simulink model "MPC"  (R2024b)
settings: Solver=ode4  StartTime=0.0  StopTime=tsim  FixedStep=baseRate  RelTol=1e-6  AbsTol=1e-6
values from neighbouring files (symbols this model uses):
  C = [cos(theta), -sin(theta) ... (first row only)    [Run_Initializer.m]    (also in plotBatch.m = quat2Rotm(q','scalarFirst'))
  camera_FOV = 40*d2r    (= 0.698131700798)    [Run_Initializer.m]
  camera_offset = [0.145, 0.087]'    [Run_Initializer.m]
  docking_face = [0 1]'    [Run_Initializer.m]
  docking_offset = [0 0 0]'    [Run_Initializer.m]
  eta = 0.7    [Run_Initializer.m]
  F_t = [kron(eye(N_h),  [zeros(2,3), eye(2), zeros(2,4)]) ... (first row only)    [Run_Initializer.m]
  f_t = [kron(ones(N_h, 1), [xLength yLength]' - edge_buffer) ... (first row only)    [Run_Initializer.m]
  F_u = [kron(eye(N_h),  [eye(3), zeros(3,6)]) ... (first row only)    [Run_Initializer.m]
  f_u = kron(ones(2*N_h, 1), u_max')    [Run_Initializer.m]
  F_v = [kron(eye(N_h),  [zeros(1,5), 1, zeros(1,3)]) ... (first row only)    [Run_Initializer.m]
  gamma = 0.95    [Run_Initializer.m]
  Gamma1_el = 0.12    [Run_Initializer.m]
  Gamma1_sh = 0.005    [Run_Initializer.m]
  Gamma1_wr = 0.025    [Run_Initializer.m]
  Gamma2_el = 5    [Run_Initializer.m]
  Gamma2_sh = 5    [Run_Initializer.m]
  Gamma2_wr = 5    [Run_Initializer.m]
  Gamma3_el = 10    [Run_Initializer.m]
  Gamma3_sh = 40    [Run_Initializer.m]
  Gamma3_wr = 40    [Run_Initializer.m]
  Gamma4_el = 0.039    [Run_Initializer.m]
  Gamma4_sh = 0.015    [Run_Initializer.m]
  Gamma4_wr = 0.029    [Run_Initializer.m]
  Gamma5_el = 800    [Run_Initializer.m]
  Gamma5_sh = 800    [Run_Initializer.m]
  Gamma5_wr = 800    [Run_Initializer.m]
  Gamma6_el = 0.000001    (= 1e-06)    [Run_Initializer.m]
  Gamma6_sh = 0.005    [Run_Initializer.m]
  Gamma6_wr = 0.02    [Run_Initializer.m]
  H = kron(eye(N_h), [R, zeros(3,6); zeros(6,3), Q])    [Run_Initializer.m]
  IBLACK = 0.1996    [unpackData.m]
  IRED = 0.1982    [unpackData.m]
  J = sum(wp*posErr + wt*angErr)    [find_transformation.m]
  Kd_elarm = 0.8    [Run_Initializer.m]
  Kd_sharm = 1.0    (= 1)    [Run_Initializer.m]
  Kd_wrarm = 0.6    [Run_Initializer.m]
  Kp_elarm = 1.2    [Run_Initializer.m]
  Kp_sharm = 1.5    [Run_Initializer.m]
  Kp_wrarm = 1.0    (= 1)    [Run_Initializer.m]
  m = m + 5    (= 4)    [unpackData.m]
  M = diag([1/m; 1/m; 1/I])    [unpackData.m]
  maxd = [d1 ... (first row only)    [Run_Initializer.m]
  mBLACK = 11.3620    (= 11.362)    [unpackData.m]
  mRED = 11.2970    (= 11.297)    [unpackData.m]
  N = size(rel,1)    [plotBatch.m]    (also in unpackData.m = 0)
  p = [0 obj.pos(k,:)]    [SparseState6DOF.m]
  PDQ = blkdiag(20*eye(3),eye(3), 20*eye(3),eye(3))    [Run_Initializer.m]
  PQ = blkdiag(20*eye(6),eye(6))    [Run_Initializer.m]
  PR = blkdiag(20*eye(3), eye(6), 0.0001*eye(3))    [Run_Initializer.m]
  PWMFreq = 5    [Run_Initializer.m]
  Q = diag([100 100 100 300 300 300])    [Run_Initializer.m]    (also in unpackData.m = blkdiag(0.0001*eye(2), 0.00001))
  R = diag([200 200 200])    [Run_Initializer.m]    (also in plotBatch.m = C3(yaw); unpackData.m = diag([6;6;6]))
  r_hold_obs = 1.1*sqrt(2)*0.3.*[1 1]    [Run_Initializer.m]
  r_hold_tar_min = [0.8; (0.3+0.05)]    [Run_Initializer.m]
  rho = 0.98    [Run_Initializer.m]
  T_d = 2    [Run_Initializer.m]
  T_max = 0.15    [Run_Initializer.m]
  Tz_lim_elarm = .1    (= 0.1)    [Run_Initializer.m]
  Tz_lim_sharm = .1    (= 0.1)    [Run_Initializer.m]
  Tz_lim_wrarm = .1    (= 0.1)    [Run_Initializer.m]
  use_LOS_constr = 1    [Run_Initializer.m]
  use_table_constr = 1    [Run_Initializer.m]
  x_BLACK_0 = [(1/3)*xLength (1/3)*yLength-0.2 280*d2r 0.01 0.005 1.88*d2r]'    [Run_Initializer.m]
  x_BLUE_0 = [0 0 0 0 0 0]'    [Run_Initializer.m]
  zeta = 10*d2r    (= 0.174532925199)    [Run_Initializer.m]
undefined symbols (not defined in the file or in its folder): a1, a2, a3, alpha, alpha_m, alpha_t, alphas, alphas_t, alphat, Am, b, b0, b1, b2, b3, baseRate, Bm, c, c1, c1t, c2, c2t, Cm, d, dataRate, DiscIntNeverNeededParam, Dm, drop_states_ARM, drop_states_BLACK, drop_states_BLUE, drop_states_RED, epsilon, epsilont, F_black_X_nominal, F_black_Y_nominal, F_blue_X_nominal, F_blue_Y_nominal, F_max, F_red_X_nominal, F_red_Y_nominal, F_thrusters_BLACK, F_thrusters_BLUE, F_thrusters_RED, gamma_I, gamma_I_t, gamma_P, gamma_P_t, home_states_BLACK, home_states_BLUE, home_states_RED, IBLUE, IDIST, IEE, init_states_BLACK, init_states_BLUE, init_states_RED, IPROX, k, K, k1 ... (+62)
libraries: simulink x33, nvidiaSharedBlocks x13, slpidlib x6, MainLibrary x5, dspsigops x3, dspinverses x3, nvidiaIMUSensorslib x1
(part 6 of 12)

== system MPC/3 - Navigation/Subsystem/QMEKF ==
  Data Store Read : DataStoreRead  DataStoreName=dt  IndexOptions=Index vector (dialog)  Indices=1  OutputSizes=1
  Data Store Read1 : DataStoreRead  DataStoreName=Red_q  IndexOptions=Index vector (dialog)  Indices=1  OutputSizes=1
  Data Store Read2 : DataStoreRead  DataStoreName=Red_x  IndexOptions=Index vector (dialog)  Indices=1  OutputSizes=1
  Data Store Read3 : DataStoreRead  DataStoreName=Vis_q  IndexOptions=Index vector (dialog)  Indices=1  OutputSizes=1
  Data Store Read4 : DataStoreRead  DataStoreName=Vis_x  IndexOptions=Index vector (dialog)  Indices=1  OutputSizes=1
  Data Store Write1 : DataStoreWrite  DataStoreName=QMEKFerror  IndexOptions=Index vector (dialog)  Indices=1  OutputSizes=1
  Data Store Write17 : DataStoreWrite  DataStoreName=QMEKFx  IndexOptions=Index vector (dialog)  Indices=1  OutputSizes=1
  Data Store Write18 : DataStoreWrite  DataStoreName=QMEKFP  IndexOptions=Index vector (dialog)  Indices=1  OutputSizes=1
  Data Store Write19 : DataStoreWrite  DataStoreName=QMEKFt  IndexOptions=Index vector (dialog)  Indices=1  OutputSizes=1
  Data Store Write2 : DataStoreWrite  DataStoreName=QMEKFNIS  IndexOptions=Index vector (dialog)  Indices=1  OutputSizes=1
  Delay : Delay  DelayLength=1  InitialCondition=PQ
  Delay1 : Delay  DelayLength=1  InitialCondition=[1;zeros(12,1)]
  MATLAB Function : MATLAB Function  TreatAsAtomicUnit=on
  MATLAB Function1 : MATLAB Function  TreatAsAtomicUnit=on
  wires:
  Delay/1 -> MATLAB Function1/7(P_prev)
  MATLAB Function1/2(P_est) -> Delay/1, Data Store Write18/1
  Delay1/1 -> MATLAB Function1/6(x_prev)
  MATLAB Function1/1(x_est) -> MATLAB Function/1(u), Delay1/1
  MATLAB Function1/3(compT) -> Data Store Write19/1
  Data Store Read/1 -> MATLAB Function1/1(dt)
  Data Store Read1/1 -> MATLAB Function1/2(RED_quat)
  Data Store Read2/1 -> MATLAB Function1/3(RED_x)
  Data Store Read3/1 -> MATLAB Function1/4(BLACK_q)
  Data Store Read4/1 -> MATLAB Function1/5(BLACK_x)
  MATLAB Function/1(out) -> Data Store Write17/1
  MATLAB Function1/5(NIS) -> Data Store Write2/1  "NIS"
  MATLAB Function1/4(y) -> Data Store Write1/1

== system MPC/3 - Navigation/Subsystem/RMEKF ==
  Data Store Read : DataStoreRead  DataStoreName=dt  IndexOptions=Index vector (dialog)  Indices=1  OutputSizes=1
  Data Store Read15 : DataStoreRead  DataStoreName=Vis_R  IndexOptions=Index vector (dialog)  Indices=1  OutputSizes=1
  Data Store Read2 : DataStoreRead  DataStoreName=Red_x  IndexOptions=Index vector (dialog)  Indices=1  OutputSizes=1
  Data Store Read3 : DataStoreRead  DataStoreName=Red_q  IndexOptions=Index vector (dialog)  Indices=1  OutputSizes=1
  Data Store Read4 : DataStoreRead  DataStoreName=Vis_x  IndexOptions=Index vector (dialog)  Indices=1  OutputSizes=1
  Data Store Write1 : DataStoreWrite  DataStoreName=RMEKFR  IndexOptions=Index vector (dialog)  Indices=1  OutputSizes=1
  Data Store Write17 : DataStoreWrite  DataStoreName=RMEKFx  IndexOptions=Index vector (dialog)  Indices=1  OutputSizes=1
  Data Store Write18 : DataStoreWrite  DataStoreName=RMEKFP  IndexOptions=Index vector (dialog)  Indices=1  OutputSizes=1
  Data Store Write19 : DataStoreWrite  DataStoreName=RMEKFt  IndexOptions=Index vector (dialog)  Indices=1  OutputSizes=1
  Data Store Write2 : DataStoreWrite  DataStoreName=RMEKFerror  IndexOptions=Index vector (dialog)  Indices=1  OutputSizes=1
  Data Store Write6 : DataStoreWrite  DataStoreName=RMEKFNIS  IndexOptions=Index vector (dialog)  Indices=1  OutputSizes=1
  Delay : Delay  DelayLength=1  InitialCondition=PR
  Delay1 : Delay  DelayLength=1  InitialCondition=zeros(9,1)
  Delay2 : Delay  DelayLength=1  InitialCondition=eye(3)
  MATLAB Function : MATLAB Function  TreatAsAtomicUnit=on
  MATLAB Function1 : MATLAB Function  TreatAsAtomicUnit=on
  MATLAB Function11 : MATLAB Function  TreatAsAtomicUnit=on
  wires:
  Delay/1 -> MATLAB Function1/8(P_prev)
  MATLAB Function1/3(P_est) -> Delay/1, Data Store Write18/1
  Delay1/1 -> MATLAB Function1/6(x_prev)
  MATLAB Function1/1(x_est) -> Delay1/1, MATLAB Function/1(x)
  MATLAB Function1/4(compT) -> Data Store Write19/1
  Data Store Read/1 -> MATLAB Function1/1(dt)
  Data Store Read3/1 -> MATLAB Function1/2(RED_yaw)
  Data Store Read2/1 -> MATLAB Function1/3(RED_x)
  Data Store Read15/1 -> MATLAB Function1/4(VIS_R)
  Data Store Read4/1 -> MATLAB Function1/5(VIS_x)
  MATLAB Function1/2(Rot_est) -> Delay2/1, Data Store Write1/1, MATLAB Function11/1(u)
  Delay2/1 -> MATLAB Function1/7(Rot_prev)
  MATLAB Function11/1(y) -> MATLAB Function/2(q)  "q"
  MATLAB Function/1(out) -> Data Store Write17/1
  MATLAB Function1/6(NIS) -> Data Store Write6/1  "NIS"
  MATLAB Function1/5(y) -> Data Store Write2/1

== system MPC/3 - Navigation/Subsystem/Representations ==
  u : Inport
  MATLAB Function : MATLAB Function  TreatAsAtomicUnit=on
  dq : Outport
  q : Outport  Port=2
  R : Outport  Port=3
  x : Outport  Port=4
  v : Outport  Port=5
  w : Outport  Port=6
  yaw : Outport  Port=7
  wires:
  u/1 -> MATLAB Function/1(u)
  MATLAB Function/1(dq) -> dq/1
  MATLAB Function/2(q) -> q/1
  MATLAB Function/3(R) -> R/1
  MATLAB Function/4(x) -> x/1
  MATLAB Function/5(v) -> v/1
  MATLAB Function/6(w) -> w/1
  MATLAB Function/7(yaw) -> yaw/1

== system MPC/3 - Navigation/Subsystem/Representations1 ==
  u : Inport
  MATLAB Function : MATLAB Function  TreatAsAtomicUnit=on
  dq : Outport
  q : Outport  Port=2
  R : Outport  Port=3
  x : Outport  Port=4
  v : Outport  Port=5
  w : Outport  Port=6
  yaw : Outport  Port=7
  wires:
  u/1 -> MATLAB Function/1(u)
  MATLAB Function/1(dq) -> dq/1
  MATLAB Function/2(q) -> q/1
  MATLAB Function/3(R) -> R/1
  MATLAB Function/4(x) -> x/1
  MATLAB Function/5(v) -> v/1
  MATLAB Function/6(w) -> w/1
  MATLAB Function/7(yaw) -> yaw/1

== system MPC/3 - Navigation/Subsystem/STDQMEKF ==
  Data Store Read : DataStoreRead  DataStoreName=dt  IndexOptions=Index vector (dialog)  Indices=1  OutputSizes=1
  Data Store Read1 : DataStoreRead  DataStoreName=Vis_dq  IndexOptions=Index vector (dialog)  Indices=1  OutputSizes=1
  Data Store Read2 : DataStoreRead  DataStoreName=Red_dq  IndexOptions=Index vector (dialog)  Indices=1  OutputSizes=1
  Data Store Write1 : DataStoreWrite  DataStoreName=STDQMEKFerror  IndexOptions=Index vector (dialog)  Indices=1  OutputSizes=1
  Data Store Write17 : DataStoreWrite  DataStoreName=STDQMEKFx  IndexOptions=Index vector (dialog)  Indices=1  OutputSizes=1
  Data Store Write18 : DataStoreWrite  DataStoreName=STDQMEKFP  IndexOptions=Index vector (dialog)  Indices=1  OutputSizes=1
  Data Store Write19 : DataStoreWrite  DataStoreName=STDQMEKFt  IndexOptions=Index vector (dialog)  Indices=1  OutputSizes=1
  Data Store Write2 : DataStoreWrite  DataStoreName=STDQMEKFNIS  IndexOptions=Index vector (dialog)  Indices=1  OutputSizes=1
  Delay : Delay  DelayLength=1  InitialCondition=PDQ
  Delay1 : Delay  DelayLength=1  InitialCondition=[1;zeros(13,1)]
  Delay2 : Delay  DelayLength=1  InitialCondition=zeros(6)
  MATLAB Function1 : MATLAB Function  TreatAsAtomicUnit=on
  MATLAB Function3 : MATLAB Function  TreatAsAtomicUnit=on
  wires:
  Delay/1 -> MATLAB Function1/5(P_prev)
  Delay1/1 -> MATLAB Function1/4(x_prev)
  MATLAB Function1/1(x_est) -> Delay1/1, MATLAB Function3/1(u)
  Data Store Read/1 -> MATLAB Function1/1(dt)
  MATLAB Function1/6(V_est) -> Delay2/1
  Delay2/1 -> MATLAB Function1/6(V_prev)
  Data Store Read2/1 -> MATLAB Function1/2(RED_dq)
  Data Store Read1/1 -> MATLAB Function1/3(VIS_dq)
  MATLAB Function1/3(compT) -> Data Store Write19/1
  MATLAB Function3/1(x) -> Data Store Write17/1
  MATLAB Function1/2(P_est) -> Delay/1, Data Store Write18/1
  MATLAB Function1/4(y) -> Data Store Write1/1
  MATLAB Function1/5(NIS) -> Data Store Write2/1

== system MPC/3 - Navigation/Subsystem/STDQMEKF1 ==
  Data Store Read : DataStoreRead  DataStoreName=dt  IndexOptions=Index vector (dialog)  Indices=1  OutputSizes=1
  Data Store Read1 : DataStoreRead  DataStoreName=Vis_dq  IndexOptions=Index vector (dialog)  Indices=1  OutputSizes=1
  Data Store Read2 : DataStoreRead  DataStoreName=Red_dq  IndexOptions=Index vector (dialog)  Indices=1  OutputSizes=1
  Data Store Write1 : DataStoreWrite  DataStoreName=STDQMEKFerror2  IndexOptions=Index vector (dialog)  Indices=1  OutputSizes=1
  Data Store Write17 : DataStoreWrite  DataStoreName=STDQMEKFx2  IndexOptions=Index vector (dialog)  Indices=1  OutputSizes=1
  Data Store Write18 : DataStoreWrite  DataStoreName=STDQMEKFP2  IndexOptions=Index vector (dialog)  Indices=1  OutputSizes=1
  Data Store Write19 : DataStoreWrite  DataStoreName=STDQMEKFt2  IndexOptions=Index vector (dialog)  Indices=1  OutputSizes=1
  Data Store Write2 : DataStoreWrite  DataStoreName=STDQMEKFNIS2  IndexOptions=Index vector (dialog)  Indices=1  OutputSizes=1
  Delay : Delay  DelayLength=1  InitialCondition=PDQ
  Delay1 : Delay  DelayLength=1  InitialCondition=[1;zeros(13,1)]
  Delay2 : Delay  DelayLength=1  InitialCondition=zeros(6)
  MATLAB Function1 : MATLAB Function  TreatAsAtomicUnit=on
  MATLAB Function3 : MATLAB Function  TreatAsAtomicUnit=on
  wires:
  Delay/1 -> MATLAB Function1/5(P_prev)
  Delay1/1 -> MATLAB Function1/4(x_prev)
  MATLAB Function1/1(x_est) -> Delay1/1, MATLAB Function3/1(u)
  Data Store Read/1 -> MATLAB Function1/1(dt)
  MATLAB Function1/6(V_est) -> Delay2/1
  Delay2/1 -> MATLAB Function1/6(V_prev)
  Data Store Read2/1 -> MATLAB Function1/2(RED_dq)
  Data Store Read1/1 -> MATLAB Function1/3(VIS_dq)
  MATLAB Function1/3(compT) -> Data Store Write19/1
  MATLAB Function3/1(x) -> Data Store Write17/1
  MATLAB Function1/2(P_est) -> Delay/1, Data Store Write18/1
  MATLAB Function1/4(y) -> Data Store Write1/1
  MATLAB Function1/5(NIS) -> Data Store Write2/1

== system MPC/3 - Navigation/Subsystem/STQMEKF ==
  Data Store Read : DataStoreRead  DataStoreName=dt  IndexOptions=Index vector (dialog)  Indices=1  OutputSizes=1
  Data Store Read1 : DataStoreRead  DataStoreName=Red_q  IndexOptions=Index vector (dialog)  Indices=1  OutputSizes=1
  Data Store Read2 : DataStoreRead  DataStoreName=Red_x  IndexOptions=Index vector (dialog)  Indices=1  OutputSizes=1
  Data Store Read3 : DataStoreRead  DataStoreName=Vis_q  IndexOptions=Index vector (dialog)  Indices=1  OutputSizes=1
  Data Store Read4 : DataStoreRead  DataStoreName=Vis_x  IndexOptions=Index vector (dialog)  Indices=1  OutputSizes=1
  Data Store Write1 : DataStoreWrite  DataStoreName=STQMEKFerror  IndexOptions=Index vector (dialog)  Indices=1  OutputSizes=1
  Data Store Write17 : DataStoreWrite  DataStoreName=STQMEKFx  IndexOptions=Index vector (dialog)  Indices=1  OutputSizes=1
  Data Store Write18 : DataStoreWrite  DataStoreName=STQMEKFP  IndexOptions=Index vector (dialog)  Indices=1  OutputSizes=1
  Data Store Write19 : DataStoreWrite  DataStoreName=STQMEKFt  IndexOptions=Index vector (dialog)  Indices=1  OutputSizes=1
  Data Store Write2 : DataStoreWrite  DataStoreName=STQMEKFNIS  IndexOptions=Index vector (dialog)  Indices=1  OutputSizes=1
  Delay : Delay  DelayLength=1  InitialCondition=PQ
  Delay1 : Delay  DelayLength=1  InitialCondition=[1;zeros(12,1)]
  Delay2 : Delay  DelayLength=1  InitialCondition=zeros(6)
  MATLAB Function1 : MATLAB Function  TreatAsAtomicUnit=on
  MATLAB Function2 : MATLAB Function  TreatAsAtomicUnit=on
  wires:
  Delay/1 -> MATLAB Function1/7(P_prev)
  MATLAB Function1/2(P_est) -> Delay/1, Data Store Write18/1
  Delay1/1 -> MATLAB Function1/6(x_prev)
  MATLAB Function1/1(x_est) -> MATLAB Function2/1(u), Delay1/1
  Data Store Read/1 -> MATLAB Function1/1(dt)
  Data Store Read1/1 -> MATLAB Function1/2(RED_quat)
  Data Store Read2/1 -> MATLAB Function1/3(RED_x)
  Data Store Read3/1 -> MATLAB Function1/4(BLACK_q)
  Data Store Read4/1 -> MATLAB Function1/5(BLACK_x)
  MATLAB Function1/6(V_est) -> Delay2/1
  Delay2/1 -> MATLAB Function1/8(V_prev)
  MATLAB Function2/1(out) -> Data Store Write17/1
  MATLAB Function1/4(y) -> Data Store Write1/1
  MATLAB Function1/5(NIS) -> Data Store Write2/1  "NIS"
  MATLAB Function1/3(compT) -> Data Store Write19/1

== system MPC/3 - Navigation/Subsystem/STQMEKF1 ==
  Data Store Read : DataStoreRead  DataStoreName=dt  IndexOptions=Index vector (dialog)  Indices=1  OutputSizes=1
  Data Store Read1 : DataStoreRead  DataStoreName=Red_q  IndexOptions=Index vector (dialog)  Indices=1  OutputSizes=1
  Data Store Read2 : DataStoreRead  DataStoreName=Red_x  IndexOptions=Index vector (dialog)  Indices=1  OutputSizes=1
  Data Store Read3 : DataStoreRead  DataStoreName=Vis_q  IndexOptions=Index vector (dialog)  Indices=1  OutputSizes=1
  Data Store Read4 : DataStoreRead  DataStoreName=Vis_x  IndexOptions=Index vector (dialog)  Indices=1  OutputSizes=1
  Data Store Write1 : DataStoreWrite  DataStoreName=STQMEKFerror2  IndexOptions=Index vector (dialog)  Indices=1  OutputSizes=1
  Data Store Write17 : DataStoreWrite  DataStoreName=STQMEKFx2  IndexOptions=Index vector (dialog)  Indices=1  OutputSizes=1
  Data Store Write18 : DataStoreWrite  DataStoreName=STQMEKFP2  IndexOptions=Index vector (dialog)  Indices=1  OutputSizes=1
  Data Store Write19 : DataStoreWrite  DataStoreName=STQMEKFt2  IndexOptions=Index vector (dialog)  Indices=1  OutputSizes=1
  Data Store Write2 : DataStoreWrite  DataStoreName=STQMEKFNIS2  IndexOptions=Index vector (dialog)  Indices=1  OutputSizes=1
  Delay : Delay  DelayLength=1  InitialCondition=PQ
  Delay1 : Delay  DelayLength=1  InitialCondition=[1;zeros(12,1)]
  Delay2 : Delay  DelayLength=1  InitialCondition=zeros(6)
  MATLAB Function1 : MATLAB Function  TreatAsAtomicUnit=on
  MATLAB Function2 : MATLAB Function  TreatAsAtomicUnit=on
  wires:
  Delay/1 -> MATLAB Function1/7(P_prev)
  MATLAB Function1/2(P_est) -> Delay/1, Data Store Write18/1
  Delay1/1 -> MATLAB Function1/6(x_prev)
  MATLAB Function1/1(x_est) -> MATLAB Function2/1(u), Delay1/1
  Data Store Read/1 -> MATLAB Function1/1(dt)
  Data Store Read1/1 -> MATLAB Function1/2(RED_quat)
  Data Store Read2/1 -> MATLAB Function1/3(RED_x)
  Data Store Read3/1 -> MATLAB Function1/4(BLACK_q)
  Data Store Read4/1 -> MATLAB Function1/5(BLACK_x)
  MATLAB Function1/6(V_est) -> Delay2/1
  Delay2/1 -> MATLAB Function1/8(V_prev)
  MATLAB Function2/1(out) -> Data Store Write17/1
  MATLAB Function1/4(y) -> Data Store Write1/1
  MATLAB Function1/5(NIS) -> Data Store Write2/1  "NIS"
  MATLAB Function1/3(compT) -> Data Store Write19/1

== system MPC/3 - Navigation/Subsystem/STRMEKF ==
  Data Store Read : DataStoreRead  DataStoreName=dt  IndexOptions=Index vector (dialog)  Indices=1  OutputSizes=1
  Data Store Read1 : DataStoreRead  DataStoreName=Vis_R  IndexOptions=Index vector (dialog)  Indices=1  OutputSizes=1
  Data Store Read2 : DataStoreRead  DataStoreName=Red_x  IndexOptions=Index vector (dialog)  Indices=1  OutputSizes=1
  Data Store Read3 : DataStoreRead  DataStoreName=Red_q  IndexOptions=Index vector (dialog)  Indices=1  OutputSizes=1
  Data Store Read4 : DataStoreRead  DataStoreName=Vis_x  IndexOptions=Index vector (dialog)  Indices=1  OutputSizes=1
  Data Store Write1 : DataStoreWrite  DataStoreName=STRMEKFR  IndexOptions=Index vector (dialog)  Indices=1  OutputSizes=1
  Data Store Write17 : DataStoreWrite  DataStoreName=STRMEKFx  IndexOptions=Index vector (dialog)  Indices=1  OutputSizes=1
  Data Store Write18 : DataStoreWrite  DataStoreName=STRMEKFP  IndexOptions=Index vector (dialog)  Indices=1  OutputSizes=1
  Data Store Write19 : DataStoreWrite  DataStoreName=STRMEKFt  IndexOptions=Index vector (dialog)  Indices=1  OutputSizes=1
  Data Store Write2 : DataStoreWrite  DataStoreName=STRMEKFerror  IndexOptions=Index vector (dialog)  Indices=1  OutputSizes=1
  Data Store Write6 : DataStoreWrite  DataStoreName=STRMEKFNIS  IndexOptions=Index vector (dialog)  Indices=1  OutputSizes=1
  Delay1 : Delay  DelayLength=1  InitialCondition=zeros(9,1)
  Delay2 : Delay  DelayLength=1  InitialCondition=PR
  Delay3 : Delay  DelayLength=1  InitialCondition=zeros(6)
  Delay4 : Delay  DelayLength=1  InitialCondition=eye(3)
  MATLAB Function : MATLAB Function  TreatAsAtomicUnit=on
  MATLAB Function1 : MATLAB Function  TreatAsAtomicUnit=on
  MATLAB Function11 : MATLAB Function  TreatAsAtomicUnit=on
  wires:
  Data Store Read/1 -> MATLAB Function1/1(dt)
  Data Store Read3/1 -> MATLAB Function1/2(RED_yaw)
  Data Store Read2/1 -> MATLAB Function1/3(RED_x)
  Data Store Read1/1 -> MATLAB Function1/4(VIS_R)
  Data Store Read4/1 -> MATLAB Function1/5(VIS_x)
  Delay2/1 -> MATLAB Function1/8(P_prev)
  Delay1/1 -> MATLAB Function1/6(x_prev)
  Delay3/1 -> MATLAB Function1/9(V_prev)
  MATLAB Function1/7(V_est) -> Delay3/1
  Delay4/1 -> MATLAB Function1/7(Rot_prev)
  MATLAB Function1/6(NIS) -> Data Store Write6/1  "NIS"
  MATLAB Function1/5(y) -> Data Store Write2/1
  MATLAB Function/1(out) -> Data Store Write17/1
  MATLAB Function1/3(P_est) -> Delay2/1, Data Store Write18/1
  MATLAB Function1/1(x_est) -> Delay1/1, MATLAB Function/1(x)
  MATLAB Function1/4(compT) -> Data Store Write19/1
  MATLAB Function1/2(Rot_est) -> Delay4/1, MATLAB Function11/1(u), Data Store Write1/1
  MATLAB Function11/1(y) -> MATLAB Function/2(q)  "q"

== system MPC/3 - Navigation/Subsystem/STRMEKF1 ==
  Data Store Read : DataStoreRead  DataStoreName=dt  IndexOptions=Index vector (dialog)  Indices=1  OutputSizes=1
  Data Store Read1 : DataStoreRead  DataStoreName=Vis_R  IndexOptions=Index vector (dialog)  Indices=1  OutputSizes=1
  Data Store Read2 : DataStoreRead  DataStoreName=Red_x  IndexOptions=Index vector (dialog)  Indices=1  OutputSizes=1
  Data Store Read3 : DataStoreRead  DataStoreName=Red_q  IndexOptions=Index vector (dialog)  Indices=1  OutputSizes=1
  Data Store Read4 : DataStoreRead  DataStoreName=Vis_x  IndexOptions=Index vector (dialog)  Indices=1  OutputSizes=1
  Data Store Write1 : DataStoreWrite  DataStoreName=STRMEKFR2  IndexOptions=Index vector (dialog)  Indices=1  OutputSizes=1
  Data Store Write17 : DataStoreWrite  DataStoreName=STRMEKFx2  IndexOptions=Index vector (dialog)  Indices=1  OutputSizes=1
  Data Store Write18 : DataStoreWrite  DataStoreName=STRMEKFP2  IndexOptions=Index vector (dialog)  Indices=1  OutputSizes=1
  Data Store Write19 : DataStoreWrite  DataStoreName=STRMEKFt2  IndexOptions=Index vector (dialog)  Indices=1  OutputSizes=1
  Data Store Write2 : DataStoreWrite  DataStoreName=STRMEKFerror2  IndexOptions=Index vector (dialog)  Indices=1  OutputSizes=1
  Data Store Write6 : DataStoreWrite  DataStoreName=STRMEKFNIS2  IndexOptions=Index vector (dialog)  Indices=1  OutputSizes=1
  Delay1 : Delay  DelayLength=1  InitialCondition=zeros(9,1)
  Delay2 : Delay  DelayLength=1  InitialCondition=PR
  Delay3 : Delay  DelayLength=1  InitialCondition=zeros(6)
  Delay4 : Delay  DelayLength=1  InitialCondition=eye(3)
  MATLAB Function : MATLAB Function  TreatAsAtomicUnit=on
  MATLAB Function1 : MATLAB Function  TreatAsAtomicUnit=on
  MATLAB Function11 : MATLAB Function  TreatAsAtomicUnit=on
  wires:
  Data Store Read/1 -> MATLAB Function1/1(dt)
  Data Store Read3/1 -> MATLAB Function1/2(RED_yaw)
  Data Store Read2/1 -> MATLAB Function1/3(RED_x)
  Data Store Read1/1 -> MATLAB Function1/4(VIS_R)
  Data Store Read4/1 -> MATLAB Function1/5(VIS_x)
  Delay2/1 -> MATLAB Function1/8(P_prev)
  Delay1/1 -> MATLAB Function1/6(x_prev)
  Delay3/1 -> MATLAB Function1/9(V_prev)
  MATLAB Function1/7(V_est) -> Delay3/1
  Delay4/1 -> MATLAB Function1/7(Rot_prev)
  MATLAB Function1/6(NIS) -> Data Store Write6/1  "NIS"
  MATLAB Function1/5(y) -> Data Store Write2/1
  MATLAB Function/1(out) -> Data Store Write17/1
  MATLAB Function1/3(P_est) -> Delay2/1, Data Store Write18/1
  MATLAB Function1/1(x_est) -> Delay1/1, MATLAB Function/1(x)
  MATLAB Function1/4(compT) -> Data Store Write19/1
  MATLAB Function1/2(Rot_est) -> Delay4/1, MATLAB Function11/1(u), Data Store Write1/1
  MATLAB Function11/1(y) -> MATLAB Function/2(q)  "q"

== system MPC/4 - Control/Default LQR Control (BLACK)/Calculate Error ==
  Desired Attitude : Inport
  Measured Attitude : Inport  Port=2
  MATLAB Function : MATLAB Function  TreatAsAtomicUnit=on
  Attitude Error : Outport
  wires:
  MATLAB Function/1(Rz_error) -> Attitude Error/1
  Desired Attitude/1 -> MATLAB Function/1(Rz_path)
  Measured Attitude/1 -> MATLAB Function/2(Rz_measured)

== system MPC/4 - Control/Default LQR Control (BLUE)/Calculate Error ==
  Desired Attitude : Inport
  Measured Attitude : Inport  Port=2
  MATLAB Function : MATLAB Function  TreatAsAtomicUnit=on
  Attitude Error : Outport
  wires:
  MATLAB Function/1(Rz_error) -> Attitude Error/1
  Desired Attitude/1 -> MATLAB Function/1(Rz_path)
  Measured Attitude/1 -> MATLAB Function/2(Rz_measured)

== system MPC/4 - Control/Default LQR Control (RED)/Calculate Error ==
  Desired Attitude : Inport
  Measured Attitude : Inport  Port=2
  MATLAB Function : MATLAB Function  TreatAsAtomicUnit=on
  Attitude Error : Outport
  wires:
  MATLAB Function/1(Rz_error) -> Attitude Error/1
  Desired Attitude/1 -> MATLAB Function/1(Rz_path)
  Measured Attitude/1 -> MATLAB Function/2(Rz_measured)

== system MPC/4 - Control/Default PD (ARM)/Passthrough for Experiment ==
  q1_desired : Inport
  q2_desired : Inport  Port=2
  q3_desired : Inport  Port=3
  Action Port : ActionPort  ActionPortLabel=else
  q1_command : Outport
  q2_command : Outport  Port=2
  q3_command : Outport  Port=3
  wires:
  q3_desired/1 -> q3_command/1
  q1_desired/1 -> q1_command/1
  q2_desired/1 -> q2_command/1

== system MPC/4 - Control/Default PD (ARM)/Simulated Position Controller ==
  q1_desired : Inport
  q2_desired : Inport  Port=2
  q3_desired : Inport  Port=3
  Action Port : ActionPort  ActionPortLabel=if(u1 == 1)
  Custom Discrete PD (Elbow) : Subsystem
  Custom Discrete PD (Shoulder) : Subsystem
  Custom Discrete PD (Wrist) : Subsystem
  Data Store Read2 : DataStoreRead  DataStoreName=ARM_Measured_States  IndexOptions=Index vector (dialog)  Indices=1  OutputSizes=1
  Demux : Demux  Outputs=[1,1,1,3]
  Saturation : Saturate  UpperLimit=Tz_lim_sharm  LowerLimit=-Tz_lim_sharm
  Saturation1 : Saturate  UpperLimit=Tz_lim_elarm  LowerLimit=-Tz_lim_elarm
  Saturation3 : Saturate  UpperLimit=Tz_lim_wrarm  LowerLimit=-Tz_lim_wrarm
  Subtract2 : Sum  Inputs=+-
  Subtract3 : Sum  Inputs=+-
  Subtract4 : Sum  Inputs=+-
  Terminator : Terminator
  q1_command : Outport
  q2_command : Outport  Port=2
  q3_command : Outport  Port=3
  wires:
  Saturation3/1 -> q3_command/1
  Subtract4/1 -> Custom Discrete PD (Wrist)/1(ey)
  Custom Discrete PD (Shoulder)/1(Fx) -> Saturation/1
  Custom Discrete PD (Elbow)/1(Fy) -> Saturation1/1
  Saturation/1 -> q1_command/1
  Subtract2/1 -> Custom Discrete PD (Shoulder)/1(ex)
  Saturation1/1 -> q2_command/1
  Custom Discrete PD (Wrist)/1(Fy) -> Saturation3/1
  Subtract3/1 -> Custom Discrete PD (Elbow)/1(ey)
  Demux/1 -> Subtract2/2
  Demux/2 -> Subtract3/2
  Demux/3 -> Subtract4/2
  q1_desired/1 -> Subtract2/1
  q2_desired/1 -> Subtract3/1
  q3_desired/1 -> Subtract4/1
  Data Store Read2/1 -> Demux/1
  Demux/4 -> Terminator/1

== system MPC/4 - Control/Default PD Control (BLACK)/Calculate Error ==
  Desired Attitude : Inport
  Measured Attitude : Inport  Port=2
  MATLAB Function : MATLAB Function  TreatAsAtomicUnit=on
  Attitude Error : Outport
  wires:
  MATLAB Function/1(Rz_error) -> Attitude Error/1
  Desired Attitude/1 -> MATLAB Function/1(Rz_path)
  Measured Attitude/1 -> MATLAB Function/2(Rz_measured)

== system MPC/4 - Control/Default PD Control (BLUE)/Calculate Error ==
  Desired Attitude : Inport
  Measured Attitude : Inport  Port=2
  MATLAB Function : MATLAB Function  TreatAsAtomicUnit=on
  Attitude Error : Outport
  wires:
  MATLAB Function/1(Rz_error) -> Attitude Error/1
  Desired Attitude/1 -> MATLAB Function/1(Rz_path)
  Measured Attitude/1 -> MATLAB Function/2(Rz_measured)

== system MPC/4 - Control/Default PD Control (RED)/CSMC ==
  In1 : Inport
  Demux : Demux  Outputs=3
  MATLAB Function : MATLAB Function  TreatAsAtomicUnit=on
  MATLAB Function1 : MATLAB Function  TreatAsAtomicUnit=on
  MATLAB Function2 : MATLAB Function  TreatAsAtomicUnit=on
  MATLAB Function3 : MATLAB Function  TreatAsAtomicUnit=on
  MATLAB Function4 : MATLAB Function  TreatAsAtomicUnit=on
  MATLAB Function5 : MATLAB Function  TreatAsAtomicUnit=on
  MATLAB Function6 : MATLAB Function  TreatAsAtomicUnit=on
  MATLAB Function7 : MATLAB Function  TreatAsAtomicUnit=on
  MATLAB Function8 : MATLAB Function  TreatAsAtomicUnit=on
  Mux : Mux  Inputs=3
  Pseudo Derivative : DiscreteTransferFcn  Numerator=[N, -N]  Denominator=[1, -1 + N*Ts]
  Pseudo Derivative1 : DiscreteTransferFcn  Numerator=[N, -N]  Denominator=[1, -1 + N*Ts]
  Pseudo Derivative2 : DiscreteTransferFcn  Numerator=[N, -N]  Denominator=[1, -1 + N*Ts]
  Saturation{,1..4} (5 alike) : Saturate  UpperLimit=epsilon  LowerLimit=-epsilon
  Saturation5 : Saturate  UpperLimit=epsilont  LowerLimit=-epsilont
  Sum : Sum  Inputs=++|
  Sum1 : Sum  Inputs=++|
  Sum2 : Sum  Inputs=++|
  Out1 : Outport
  wires:
  Demux/1 -> MATLAB Function2/1(q1), Pseudo Derivative/1
  Pseudo Derivative/1 -> MATLAB Function2/2(q2), MATLAB Function1/1(q2)
  Sum/1 -> Mux/1
  MATLAB Function/1(u) -> Saturation1/1
  MATLAB Function1/1(u) -> Saturation/1
  MATLAB Function2/1(phi) -> MATLAB Function/1(phi)
  Saturation/1 -> Sum/2
  Saturation1/1 -> Sum/1
  Saturation2/1 -> Sum1/2
  MATLAB Function5/1(phi) -> MATLAB Function3/1(phi)
  Saturation3/1 -> Sum1/1
  Demux/2 -> MATLAB Function5/1(q1), Pseudo Derivative1/1
  Pseudo Derivative1/1 -> MATLAB Function4/1(q2), MATLAB Function5/2(q2)
  MATLAB Function4/1(u) -> Saturation2/1
  MATLAB Function3/1(u) -> Saturation3/1
  Sum1/1 -> Mux/2
  Demux/3 -> Pseudo Derivative2/1, MATLAB Function8/1(q1)
  MATLAB Function7/1(u) -> Saturation4/1
  Saturation4/1 -> Sum2/2
  Saturation5/1 -> Sum2/1
  Pseudo Derivative2/1 -> MATLAB Function7/1(q2), MATLAB Function8/2(q2)
  MATLAB Function8/1(phi) -> MATLAB Function6/1(phi)
  MATLAB Function6/1(u) -> Saturation5/1
  Sum2/1 -> Mux/3
  Mux/1 -> Out1/1
  In1/1 -> Demux/1

== system MPC/4 - Control/Default PD Control (RED)/Calculate Error ==
  Desired Attitude : Inport
  Measured Attitude : Inport  Port=2
  MATLAB Function : MATLAB Function  TreatAsAtomicUnit=on
  Attitude Error : Outport
  wires:
  MATLAB Function/1(Rz_error) -> Attitude Error/1
  Desired Attitude/1 -> MATLAB Function/1(Rz_path)
  Measured Attitude/1 -> MATLAB Function/2(Rz_measured)

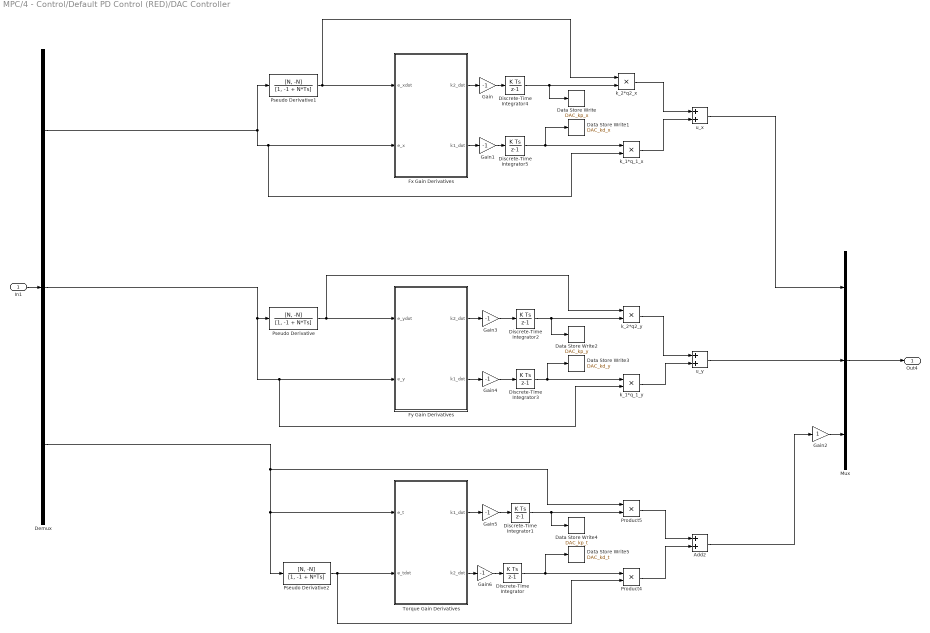
== system MPC/4 - Control/Default PD Control (RED)/DAC Controller ==
  In1 : Inport
  Add2 : Sum
  Data Store Write : DataStoreWrite  DataStoreName=DAC_kp_x  IndexOptions=Index vector (dialog)  Indices=1  OutputSizes=1
  Data Store Write1 : DataStoreWrite  DataStoreName=DAC_kd_x  IndexOptions=Index vector (dialog)  Indices=1  OutputSizes=1
  Data Store Write2 : DataStoreWrite  DataStoreName=DAC_kp_y  IndexOptions=Index vector (dialog)  Indices=1  OutputSizes=1
  Data Store Write3 : DataStoreWrite  DataStoreName=DAC_kd_y  IndexOptions=Index vector (dialog)  Indices=1  OutputSizes=1
  Data Store Write4 : DataStoreWrite  DataStoreName=DAC_kp_t  IndexOptions=Index vector (dialog)  Indices=1  OutputSizes=1
  Data Store Write5 : DataStoreWrite  DataStoreName=DAC_kd_t  IndexOptions=Index vector (dialog)  Indices=1  OutputSizes=1
  Demux : Demux  Outputs=3
  Discrete-Time Integrator : DiscreteIntegrator  InitialCondition=k_2_t_0  SampleTime=-1  ICPrevOutput=DiscIntNeverNeededParam  ICPrevScaledInput=DiscIntNeverNeededParam
  Discrete-Time Integrator1 : DiscreteIntegrator  InitialCondition=k_1_t_0  SampleTime=-1  ICPrevOutput=DiscIntNeverNeededParam  ICPrevScaledInput=DiscIntNeverNeededParam
  Discrete-Time Integrator2 : DiscreteIntegrator  InitialCondition=k_2_0  SampleTime=-1  ICPrevOutput=DiscIntNeverNeededParam  ICPrevScaledInput=DiscIntNeverNeededParam
  Discrete-Time Integrator3 : DiscreteIntegrator  InitialCondition=k_1_0  SampleTime=-1  ICPrevOutput=DiscIntNeverNeededParam  ICPrevScaledInput=DiscIntNeverNeededParam
  Discrete-Time Integrator4 : DiscreteIntegrator  InitialCondition=k_2_0  SampleTime=-1  ICPrevOutput=DiscIntNeverNeededParam  ICPrevScaledInput=DiscIntNeverNeededParam
  Discrete-Time Integrator5 : DiscreteIntegrator  InitialCondition=k_1_0  SampleTime=-1  ICPrevOutput=DiscIntNeverNeededParam  ICPrevScaledInput=DiscIntNeverNeededParam
  Fx Gain Derivatives : MATLAB Function  TreatAsAtomicUnit=on
  Fy Gain Derivatives : MATLAB Function  TreatAsAtomicUnit=on
  Gain{,1,3..6} (6 alike) : Gain  Gain=-1
  Gain2 : Gain
  Mux : Mux  Inputs=3
  Product4 : Product
  Product5 : Product
  Pseudo Derivative : DiscreteTransferFcn  Numerator=[N, -N]  Denominator=[1, -1 + N*Ts]
  Pseudo Derivative1 : DiscreteTransferFcn  Numerator=[N, -N]  Denominator=[1, -1 + N*Ts]
  Pseudo Derivative2 : DiscreteTransferFcn  Numerator=[N, -N]  Denominator=[1, -1 + N*Ts]
  Torque Gain Derivatives : MATLAB Function  TreatAsAtomicUnit=on
  k_1*q_1_x : Product
  k_1*q_1_y : Product
  k_2*q2_x : Product
  k_2*q2_y : Product
  u_x : Sum
  u_y : Sum
  Out4 : Outport
  wires:
  Add2/1 -> Gain2/1
  u_y/1 -> Mux/2
  Pseudo Derivative/1 -> k_2*q2_y/1, Fy Gain Derivatives/1(e_ydot)
  Demux/2 -> Fy Gain Derivatives/2(e_y), k_1*q_1_y/2, Pseudo Derivative/1
  k_2*q2_y/1 -> u_y/1
  Fy Gain Derivatives/2(k1_dot) -> Gain4/1
  k_1*q_1_y/1 -> u_y/2
  Fy Gain Derivatives/1(k2_dot) -> Gain3/1
  Torque Gain Derivatives/1(k1_dot) -> Gain5/1
  Pseudo Derivative2/1 -> Torque Gain Derivatives/2(e_tdot), Product4/2
  Product5/1 -> Add2/1
  Product4/1 -> Add2/2
  Torque Gain Derivatives/2(k2_dot) -> Gain6/1
  Demux/1 -> k_1*q_1_x/2, Fx Gain Derivatives/2(e_x), Pseudo Derivative1/1
  Pseudo Derivative1/1 -> k_2*q2_x/1, Fx Gain Derivatives/1(e_xdot)
  k_1*q_1_x/1 -> u_x/2
  u_x/1 -> Mux/1
  k_2*q2_x/1 -> u_x/1
  Demux/3 -> Torque Gain Derivatives/1(e_t), Pseudo Derivative2/1, Product5/1
  In1/1 -> Demux/1
  Mux/1 -> Out4/1
  Gain2/1 -> Mux/3
  Discrete-Time Integrator2/1 -> Data Store Write2/1, k_2*q2_y/2
  Discrete-Time Integrator5/1 -> Data Store Write1/1, k_1*q_1_x/1
  Discrete-Time Integrator4/1 -> Data Store Write/1, k_2*q2_x/2
  Discrete-Time Integrator1/1 -> Data Store Write4/1, Product5/2
  Fx Gain Derivatives/1(k2_dot) -> Gain/1
  Fx Gain Derivatives/2(k1_dot) -> Gain1/1
  Gain/1 -> Discrete-Time Integrator4/1
  Gain1/1 -> Discrete-Time Integrator5/1
  Gain3/1 -> Discrete-Time Integrator2/1
  Gain4/1 -> Discrete-Time Integrator3/1
  Gain5/1 -> Discrete-Time Integrator1/1
  Gain6/1 -> Discrete-Time Integrator/1
  Discrete-Time Integrator3/1 -> Data Store Write3/1, k_1*q_1_y/1
  Discrete-Time Integrator/1 -> Data Store Write5/1, Product4/1

== system MPC/4 - Control/Default PD Control (RED)/Diff ==
  In1 : Inport
  In2 : Inport  Port=2
  Demux : Demux  Outputs=3
  Demux1 : Demux  Outputs=3
  Hough Control : Subsystem
      settings: PortSchema="{\"entries\":[{\"content\":{\"sides\":[{\"content\":{\"connectorIds\":[\"In1\"]},\"type\":\"ConnectorPlacement.EquallySpacedRectSide\",\"uuid\":\"a8dcddb7-9836-4673-8356-a3c89c9502b3\"},{\"content\":{\"connectorIds\":[\"Out1\"],\"side\":\"RIGHT\"},\"type\":\"ConnectorPlacement.EquallySpacedRectSide\",\"uuid\":\"2c97d3bb-11f9-4ba2-b448-09694ac8e6f8\"},{\"content\":{\"side\":\"TOP\"},\"type\":\"ConnectorPlacement.EquallySpacedRectSide\",\"uuid\":\"bc41882c-3443-497d-b6f8-69c8cbf4c339\"},{\"content\":{\"connectorIds\":[\"In2\"],\"side\":\"BOTTOM\"},\"type\":\"ConnectorPlacement.EquallySpacedRectSide\",\"uuid\":\"14b1077a-07d2-46a7-87f1-61ebe292854a\"}]},\"type\":\"ConnectorPlacement.EquallySpacedConnector\",\"uuid\":\"2f9ed5e7-457a-4e66-9582-5133e2ff8cc8\"}],\"packageUris\":[\"http://schema.mathworks.com/mf0/Connector/R2020b\"],\"version\":\"1.0\"}"
  Mux : Mux  Inputs=3
  Sum : Sum  Inputs=|+-
  Sum1 : Sum  Inputs=|+-
  u : Outport
  wires:
  In1/1 -> Demux/1
  Demux/2 -> Sum/1
  Demux/1 -> Sum1/1
  In2/1 -> Demux1/1
  Demux1/1 -> Sum1/2
  Demux1/2 -> Sum/2
  Demux/3 -> Hough Control/1(Ref)
  Demux1/3 -> Hough Control/2(Act)
  Hough Control/1(Err) -> Mux/3
  Sum/1 -> Mux/2
  Sum1/1 -> Mux/1
  Mux/1 -> u/1

== system MPC/4 - Control/Default PD Control (RED)/H_inf ==
  In1 : Inport
  Demux : Demux  Outputs=3
  Discrete State-Space : DiscreteStateSpace  A=K.A  B=K.B  C=K.C  D=K.D  SampleTime=-1
  Discrete State-Space1 : DiscreteStateSpace  A=K_t.A  B=K_t.B  C=K_t.C  D=K_t.D  SampleTime=-1
  Discrete State-Space2 : DiscreteStateSpace  A=K.A  B=K.B  C=K.C  D=K.D  SampleTime=-1
  Mux : Mux  Inputs=3
  Out1 : Outport
  wires:
  In1/1 -> Demux/1
  Mux/1 -> Out1/1
  Demux/3 -> Discrete State-Space1/1
  Discrete State-Space1/1 -> Mux/3
  Demux/1 -> Discrete State-Space/1
  Discrete State-Space/1 -> Mux/1
  Demux/2 -> Discrete State-Space2/1
  Discrete State-Space2/1 -> Mux/2

== system MPC/4 - Control/Default PD Control (RED)/Homo ==
  In1 : Inport
  Demux : Demux  Outputs=3
  MATLAB Function : MATLAB Function  TreatAsAtomicUnit=on
  MATLAB Function1 : MATLAB Function  TreatAsAtomicUnit=on
  MATLAB Function2 : MATLAB Function  TreatAsAtomicUnit=on
  MATLAB Function3 : MATLAB Function  TreatAsAtomicUnit=on
  MATLAB Function4 : MATLAB Function  TreatAsAtomicUnit=on
  MATLAB Function5 : MATLAB Function  TreatAsAtomicUnit=on
  Mux : Mux  Inputs=3
  Pseudo Derivative : DiscreteTransferFcn  Numerator=[N, -N]  Denominator=[1, -1 + N*Ts]
  Pseudo Derivative1 : DiscreteTransferFcn  Numerator=[N, -N]  Denominator=[1, -1 + N*Ts]
  Pseudo Derivative2 : DiscreteTransferFcn  Numerator=[N, -N]  Denominator=[1, -1 + N*Ts]
  Sum : Sum  Inputs=++|
  Sum1 : Sum  Inputs=++|
  Sum2 : Sum  Inputs=++|
  Out1 : Outport
  wires:
  Demux/1 -> Pseudo Derivative/1, MATLAB Function/1(q1)
  Pseudo Derivative/1 -> MATLAB Function1/1(q2)
  Sum/1 -> Mux/1
  MATLAB Function/1(u) -> Sum/1
  MATLAB Function1/1(u) -> Sum/2
  Pseudo Derivative1/1 -> MATLAB Function3/1(q2)
  Sum1/1 -> Mux/2
  MATLAB Function3/1(u) -> Sum1/2
  Demux/2 -> MATLAB Function2/1(q1), Pseudo Derivative1/1
  MATLAB Function2/1(u) -> Sum1/1
  Demux/3 -> MATLAB Function4/1(q1), Pseudo Derivative2/1
  Pseudo Derivative2/1 -> MATLAB Function5/1(q2)
  MATLAB Function5/1(u) -> Sum2/2
  MATLAB Function4/1(u) -> Sum2/1
  Sum2/1 -> Mux/3
  Mux/1 -> Out1/1
  In1/1 -> Demux/1

== system MPC/4 - Control/Default PD Control (RED)/LQR ==
  In1 : Inport
  Constant : Constant  Value=k
  Demux : Demux  Outputs=3
  MATLAB Function : MATLAB Function  TreatAsAtomicUnit=on
  Pseudo Derivative : DiscreteTransferFcn  Numerator=[N, -N]  Denominator=[1, -1 + N*Ts]
  Pseudo Derivative1 : DiscreteTransferFcn  Numerator=[N, -N]  Denominator=[1, -1 + N*Ts]
  Pseudo Derivative2 : DiscreteTransferFcn  Numerator=[N, -N]  Denominator=[1, -1 + N*Ts]
  Out1 : Outport
  wires:
  Constant/1 -> MATLAB Function/1(k)
  MATLAB Function/1(u) -> Out1/1
  Demux/3 -> Pseudo Derivative2/1, MATLAB Function/6(q1_t)
  Demux/2 -> Pseudo Derivative1/1, MATLAB Function/4(q1_y)
  Demux/1 -> Pseudo Derivative/1, MATLAB Function/2(q1_x)
  Pseudo Derivative2/1 -> MATLAB Function/7(q2_t)
  Pseudo Derivative/1 -> MATLAB Function/3(q2_x)
  Pseudo Derivative1/1 -> MATLAB Function/5(q2_y)
  In1/1 -> Demux/1

== system MPC/4 - Control/Default PD Control (RED)/Min Energy ==
  In1 : Inport
  Clock : Clock
  Clock1 : Clock
  Clock2 : Clock
  Demux : Demux  Outputs=3
  MATLAB Function : MATLAB Function  TreatAsAtomicUnit=on
  MATLAB Function1 : MATLAB Function  TreatAsAtomicUnit=on
  MATLAB Function2 : MATLAB Function  TreatAsAtomicUnit=on
  Mux : Mux  Inputs=3
  Pseudo Derivative : DiscreteTransferFcn  Numerator=[N, -N]  Denominator=[1, -1 + N*Ts]
  Pseudo Derivative1 : DiscreteTransferFcn  Numerator=[N, -N]  Denominator=[1, -1 + N*Ts]
  Pseudo Derivative2 : DiscreteTransferFcn  Numerator=[N, -N]  Denominator=[1, -1 + N*Ts]
  Subsystem : Subsystem
  Subsystem1 : Subsystem
  Subsystem2 : Subsystem
  Sum : Sum  Inputs=|++
  Sum1 : Sum  Inputs=|++
  Sum2 : Sum  Inputs=|++
  Out1 : Outport
  wires:
  Demux/2 -> Subsystem1/2(u), Pseudo Derivative1/1, MATLAB Function/1(q1)
  Pseudo Derivative1/1 -> MATLAB Function/2(q2)
  Clock/1 -> MATLAB Function/3(t)
  MATLAB Function/1(u) -> Sum1/1
  Clock1/1 -> MATLAB Function1/3(t)
  Pseudo Derivative/1 -> MATLAB Function1/2(q2)
  MATLAB Function1/1(u) -> Sum/1
  Demux/1 -> Subsystem/2(u), MATLAB Function1/1(q1), Pseudo Derivative/1
  Clock2/1 -> MATLAB Function2/3(t)
  Pseudo Derivative2/1 -> MATLAB Function2/2(q2)
  MATLAB Function2/1(u) -> Sum2/1
  Demux/3 -> Subsystem2/2(u), Pseudo Derivative2/1, MATLAB Function2/1(q1)
  Mux/1 -> Out1/1
  In1/1 -> Demux/1
  MATLAB Function1/2(dt) -> Subsystem/1(In2)
  Sum/1 -> Mux/1
  Subsystem/1(Out1) -> Sum/2
  MATLAB Function/2(dt) -> Subsystem1/1(dt)
  Sum1/1 -> Mux/2
  Subsystem1/1(Out1) -> Sum1/2
  Sum2/1 -> Mux/3
  Subsystem2/1(Out1) -> Sum2/2
  MATLAB Function2/2(dt) -> Subsystem2/1(dt)

== system MPC/4 - Control/Default PD Control (RED)/Minimum Time Controller ==
  In1 : Inport
  Demux : Demux  Outputs=3
  Gain : Gain  Gain=F_max
  Gain1 : Gain  Gain=F_max
  Gain2 : Gain  Gain=T_max
  MATLAB Function : MATLAB Function  TreatAsAtomicUnit=on
  MATLAB Function1 : MATLAB Function  TreatAsAtomicUnit=on
  MATLAB Function2 : MATLAB Function  TreatAsAtomicUnit=on
  MATLAB Function3 : MATLAB Function  TreatAsAtomicUnit=on
  MATLAB Function4 : MATLAB Function  TreatAsAtomicUnit=on
  MATLAB Function5 : MATLAB Function  TreatAsAtomicUnit=on
  Mux : Mux  Inputs=3
  Pseudo Derivative : DiscreteTransferFcn  Numerator=[N, -N]  Denominator=[1, -1 + N*Ts]
  Pseudo Derivative1 : DiscreteTransferFcn  Numerator=[N, -N]  Denominator=[1, -1 + N*Ts]
  Pseudo Derivative2 : DiscreteTransferFcn  Numerator=[N, -N]  Denominator=[1, -1 + N*Ts]
  Out1 : Outport
  wires:
  Demux/1 -> MATLAB Function/1(q_1), MATLAB Function3/1(q_1), Pseudo Derivative/1
  Demux/3 -> Pseudo Derivative2/1, MATLAB Function2/1(q_1), MATLAB Function5/1(q_1)
  Pseudo Derivative/1 -> MATLAB Function/2(q_2)
  Demux/2 -> Pseudo Derivative1/1, MATLAB Function4/1(q_1), MATLAB Function1/1(q_1)
  Pseudo Derivative1/1 -> MATLAB Function1/2(q_2)
  Pseudo Derivative2/1 -> MATLAB Function2/2(q_2)
  MATLAB Function/1(sign_Argument) -> MATLAB Function3/2(sign_Argument)
  MATLAB Function1/1(sign_Argument) -> MATLAB Function4/2(sign_Argument)
  MATLAB Function2/1(sign_Argument) -> MATLAB Function5/2(sign_Argument)
  MATLAB Function3/1(u_max_product) -> Gain/1
  Gain/1 -> Mux/1
  MATLAB Function4/1(u_max_product) -> Gain1/1
  Gain1/1 -> Mux/2
  MATLAB Function5/1(u_max_product) -> Gain2/1
  Gain2/1 -> Mux/3
  In1/1 -> Demux/1
  Mux/1 -> Out1/1
